simulink model "dx_com_debugging"  (Simulink 7.9)
settings: Solver=ode45  StartTime=0.0  StopTime=inf  RelTol=1e-3
libraries: utility x1
settings Model: Creator=jorhabib  LastModifiedBy=jorhabib

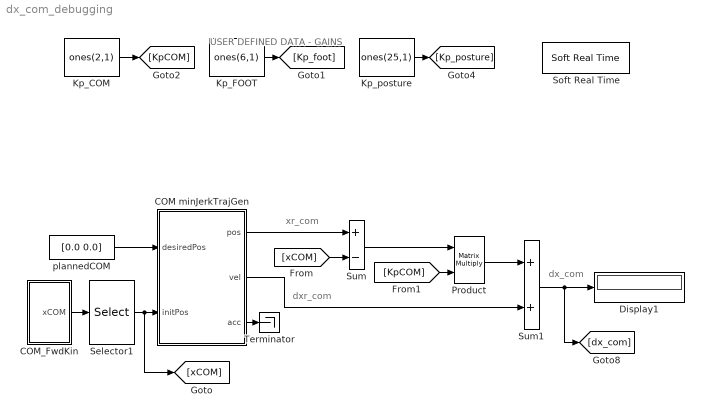
== system dx_com_debugging ==
  note: USER DEFINED DATA - GAINS
  note: xr_com
  note: dx_com
  note: dxr_com
  COM minJerkTrajGen : Subsystem
  COM_FwdKin : Subsystem
  Display1 : Display
  Kp_COM : Constant  Value=ones(2,1)
  Kp_FOOT : Constant  Value=ones(6,1)
  Kp_posture : Constant  Value=ones(25,1)
  Product : Product  Multiplication=Matrix(*)  RndMeth=Zero
  Selector1 : Selector  IndexMode=Zero-based  InputPortWidth=7  IndexOptions=Index vector (dialog)  Indices=[0:1]  OutputSizes=1
  Soft Real Time : utility/Soft Real Time  x=0.1
  Sum : Sum  Inputs=+-
  Sum1 : Sum
  Terminator : Terminator
  plannedCOM : Constant  Value=[0.0 0.0]
  wires:
  Kp_COM/1 -> [KpCOM]
  Kp_FOOT/1 -> [Kp_foot]
  Kp_posture/1 -> [Kp_posture]
  plannedCOM/1 -> COM minJerkTrajGen/1(desiredPos)
  COM minJerkTrajGen/1(pos) -> Sum/1
  COM minJerkTrajGen/3(acc) -> Terminator/1
  [xCOM] -> Sum/2
  Sum/1 -> Product/1
  [KpCOM] -> Product/2
  Product/1 -> Sum1/1
  COM minJerkTrajGen/2(vel) -> Sum1/2
  Sum1/1 -> [dx_com], Display1/1
  COM_FwdKin/1(xCOM) -> Selector1/1
  Selector1/1 -> [xCOM], COM minJerkTrajGen/2(initPos)

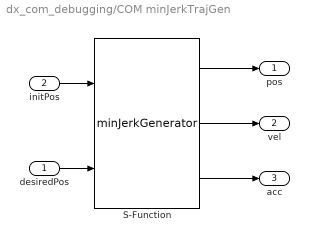
== system dx_com_debugging/COM minJerkTrajGen ==
  desiredPos : Inport
  initPos : Inport  Port=2
  S-Function : S-Function  FunctionName=minJerkGenerator  Parameters=dim, rate, tt  EnableBusSupport=off  mask{dim=2, rate=10, tt=4}
      mask prompts: dim "Trajectory dimension (int)"; rate "Simulation rate (int) [ms]"; tt "Trajectory time [s]"
  pos : Outport
  vel : Outport  Port=2
  acc : Outport  Port=3
  wires:
  S-Function/2 -> vel/1
  S-Function/1 -> pos/1
  S-Function/3 -> acc/1
  initPos/1 -> S-Function/1
  desiredPos/1 -> S-Function/2

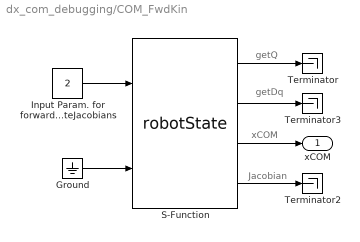
== system dx_com_debugging/COM_FwdKin ==
  note: Jacobian
  note: getQ
  note: xCOM
  note: getDq
  Ground : Ground
  "Input Param. for forwardKinematics and  computeJacobians " : Constant  Value=2  OutDataTypeStr=int8
  S-Function : S-Function  FunctionName=robotState  Parameters=val,robotname,localname  EnableBusSupport=off  mask{val=2, robotname='icubSim', localname='robotState'}
      mask prompts: val "Value"; robotname "Robot Name (icub - icubSim)"; localname "Module Name"
  Terminator : Terminator
  Terminator2 : Terminator
  Terminator3 : Terminator
  xCOM : Outport
  wires:
  Ground/1 -> S-Function/2
  S-Function/4 -> Terminator2/1
  "Input Param. for forwardKinematics and  computeJacobians "/1 -> S-Function/1
  S-Function/3 -> xCOM/1
  S-Function/1 -> Terminator/1
  S-Function/2 -> Terminator3/1
